simulink model "Device_B"  (R2025b)
settings: Solver=FixedStepAuto  StartTime=0.0  StopTime=10.0  RelTol=1e-3
undefined symbols (not defined in the file): bbb, Data_Display, Data_Display1, Data_Input2, Method_Select
libraries: androiduilib x4, dspxfrm3 x2, androidaudiovideolib x1, dspadpt3 x1, androidcommunicationlib x1
settings Model: Creator=chinm  LastModifiedBy=Windows
settings OptimizationCC: DefaultParameterBehavior=Inlined  EnhancedBackFolding=on  PassReuseOutputArgsAs=Individual arguments  ZeroExternalMemoryAtStartup=off  ZeroInternalMemoryAtStartup=off  MaxStackSize=64  OptimizeBlockOrder=speed  DifferentSizesBufferReuse=on  OptimizationCustomize=off  EfficientTunableParamExpr=on
settings DebuggingCC: ParameterTunabilityLossMsg=error
settings HardwareCC: ProdBitPerPointer=32.0  ProdBitPerSizeT=32.0  ProdBitPerPtrDiffT=32.0  ProdLargestAtomicInteger=Long  ProdLargestAtomicFloat=Double  ProdWordSize=32.0  ProdHWDeviceType=ARM Compatible->ARM Cortex-A (32-bit)
settings SFSimCC: MATLABDynamicMemAlloc=off
settings RTWCC: SystemTargetFile=ert.tlc  HardwareBoard=Android Device  TLCOptions="-aInlineSetEventsForThisBaseRateFcn=TLC_FALSE -aSuppressMultiTaskScheduler=TLC_FALSE  -aRateBasedStepFcn=0"  TemplateMakefile=ert_default_tmf  RTWVerbose=off  Toolchain=Android SDK/NDK Tools  GPUComputeCapability=3.5  Description=Embedded Coder
settings CodeAppCC: ForceParamTrailComments=on  IgnoreCustomStorageClasses=off  OperatorAnnotations=on  SimulinkDataObjDesc=on  SFDataObjDesc=on  InsertBlockDesc=on

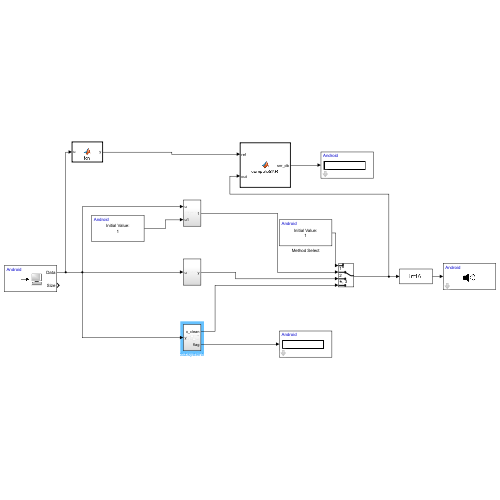
[thumbnail: Simulink's stored preview of the top-level diagram]
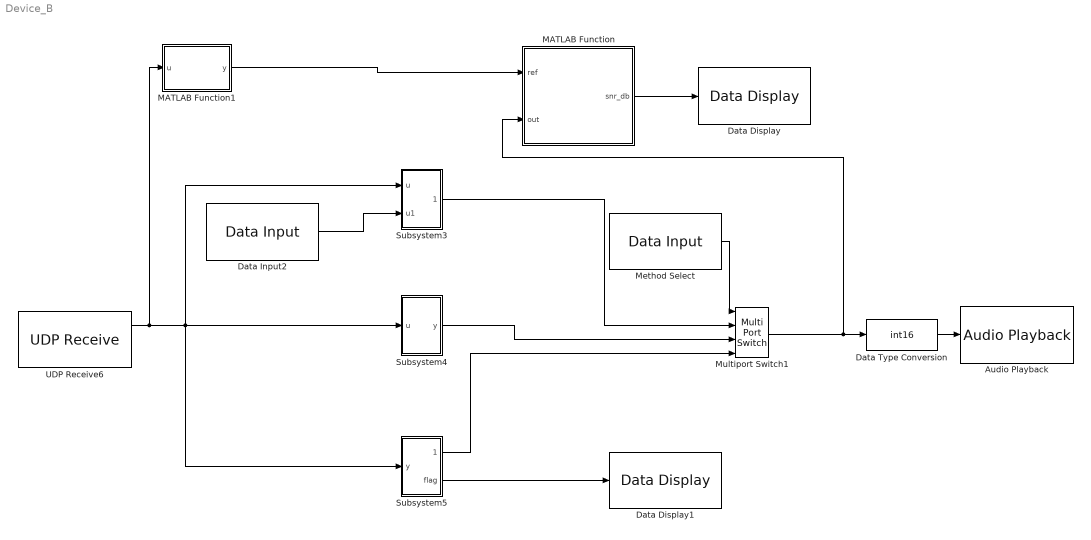
== system Device_B ==
  Audio Playback : androidaudiovideolib/Audio Playback  SampleFreq=8000  AudioSamplingFreq=8000  SampleTime=0.1  DeviceStr=0  QueueDuration=0  BlockPlatform=Android
  Data Display : androiduilib/Data Display  DataDisplayId=bbb/Data_Display  Format=Float  Precision=6  SimulateUsing=Code generation  blockPlatform=Android
  Data Display1 : androiduilib/Data Display  DataDisplayId=bbb/Data_Display1  Format=Float  Precision=6  SimulateUsing=Code generation  blockPlatform=Android
  Data Input2 : androiduilib/Data Input  isCharVector=off  Value=1.0  CharVector=Hello World  OutputDataType=int8  maxCharVectorSize=100  DataInputId=bbb/Data_Input2  SampleTime=1
  Data Type Conversion : DataTypeConversion  OutDataTypeStr=int16  SaturateOnIntegerOverflow=off  RndMeth=Floor
  MATLAB Function : MATLAB Function  TreatAsAtomicUnit=on
  MATLAB Function1 : MATLAB Function  TreatAsAtomicUnit=on
  Method Select : androiduilib/Data Input  isCharVector=off  Value=1  CharVector=Hello World  OutputDataType=int8  maxCharVectorSize=100  DataInputId=bbb/Method_Select  SampleTime=1
  Multiport Switch1 : MultiPortSwitch  DataPortOrder=Specify indices  OutDataTypeStr=double  SaturateOnIntegerOverflow=off  InputSameDT=off
  Subsystem3 : Subsystem
  Subsystem4 : Subsystem
  Subsystem5 : Subsystem
  UDP Receive6 : androidcommunicationlib/UDP Receive  localURL='0.0.0.0'  localPort=25070  remoteURL='0.0.0.0'  remotePort=-1  recvBufferSize=8192  signalDatatype=double  dims=1024  isVarSize=off  showBlockingTime=off  blockingTime=0  sampletime=0.032  blockPlatform=Android
  wires:
  Method Select/1 -> Multiport Switch1/1
  Data Input2/1 -> Subsystem3/2(u1)
  MATLAB Function/1(snr_db) -> Data Display/1
  Subsystem3/1(Out1) -> Multiport Switch1/2
  Multiport Switch1/1 -> MATLAB Function/2(out), Data Type Conversion/1
  UDP Receive6/1 -> MATLAB Function1/1(u), Subsystem4/1(u), Subsystem3/1(u), Subsystem5/1(y)
  Subsystem5/1(x_clean) -> Multiport Switch1/4
  Subsystem5/2(flag) -> Data Display1/1
  Subsystem4/1(y) -> Multiport Switch1/3
  MATLAB Function1/1(y) -> MATLAB Function/1(ref)
  Data Type Conversion/1 -> Audio Playback/1

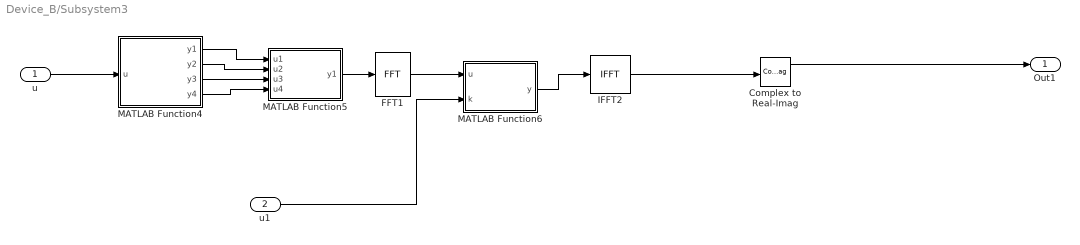
== system Device_B/Subsystem3 ==
  u : Inport
  u1 : Inport  Port=2
  Complex to Real-Imag : ComplexToRealImag
  FFT1 : dspxfrm3/FFT  FFTImplementation=Auto  CompMethod=Table lookup  TableOpt=NEW  TableOptActive=Speed  BitRevOrder=off  Normalize=off  InheritFFTLength=on  FFTLength=64  WrapInput=on  roundingMode=Ceiling  overflowMode=off  firstCoeffDataTypeStr=Inherit: Same word length as input  firstCoeffLastDataTypeStr=Inherit: Same word length as input  outputMin=[]  outputMax=[]
      settings: LockScale=on
  IFFT2 : dspxfrm3/IFFT  FFTImplementation=Auto  CompMethod=Table lookup  TableOpt=NEW  TableOptActive=Speed  BitRevOrder=off  cs_in=off  Normalize=on  InheritFFTLength=on  FFTLength=64  WrapInput=on  mode=Real  outSamplingMode=Sample based  roundingMode=Ceiling  overflowMode=off  firstCoeffDataTypeStr=Inherit: Same word length as input  firstCoeffLastDataTypeStr=Inherit: Same word length as input  outputMin=[]  outputMax=[]
  MATLAB Function4 : MATLAB Function  TreatAsAtomicUnit=on
  MATLAB Function5 : MATLAB Function  TreatAsAtomicUnit=on
  MATLAB Function6 : MATLAB Function  TreatAsAtomicUnit=on
  Out1 : Outport
  wires:
  Complex to Real-Imag/1 -> Out1/1
  IFFT2/1 -> Complex to Real-Imag/1
  MATLAB Function4/4(y4) -> MATLAB Function5/4(u4)
  u1/1 -> MATLAB Function6/2(k)
  MATLAB Function4/1(y1) -> MATLAB Function5/1(u1)
  MATLAB Function4/3(y3) -> MATLAB Function5/3(u3)
  MATLAB Function4/2(y2) -> MATLAB Function5/2(u2)
  MATLAB Function5/1(y1) -> FFT1/1
  MATLAB Function6/1(y) -> IFFT2/1
  u/1 -> MATLAB Function4/1(u)
  FFT1/1 -> MATLAB Function6/1(u)

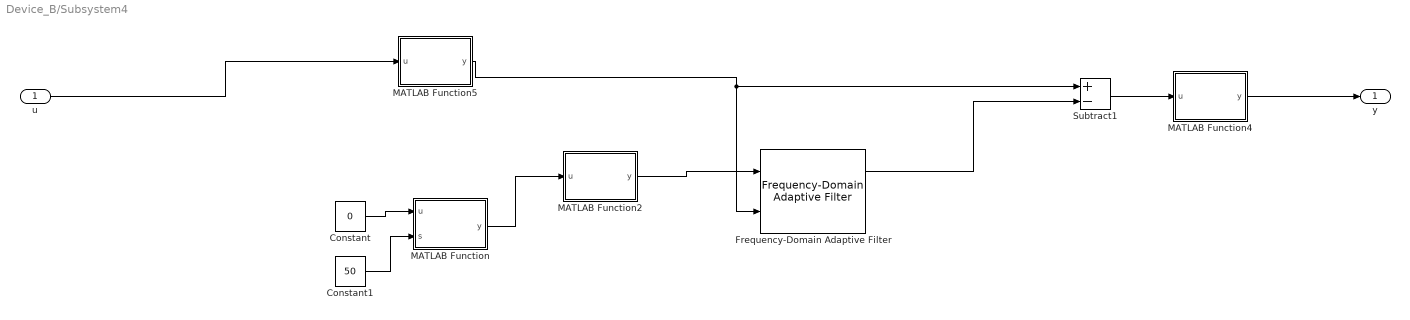
== system Device_B/Subsystem4 ==
  u : Inport
  Constant : Constant  Value=0  OutDataTypeStr=double
  Constant1 : Constant  Value=50
  Frequency-Domain Adaptive Filter : dspadpt3/Frequency-Domain Adaptive Filter  Method=Constrained FDAF  Length=32  BlockLength=32  StepSizePort=off  StepSize=1  LeakageFactorPort=off  LeakageFactor=1  AveragingFactorPort=off  AveragingFactor=0.9  OffsetPort=off  InitialPower=1  InitialCoefficients=0  AdaptPort=off  ResetPort=off  FFTCoefficientsPort=off  SimulateUsing=Interpreted execution  Offset=0
  MATLAB Function : MATLAB Function  TreatAsAtomicUnit=on
  MATLAB Function2 : MATLAB Function  TreatAsAtomicUnit=on
  MATLAB Function4 : MATLAB Function  TreatAsAtomicUnit=on
  MATLAB Function5 : MATLAB Function  TreatAsAtomicUnit=on
  Subtract1 : Sum  Inputs=+-
  y : Outport
  wires:
  MATLAB Function5/1(y) -> Frequency-Domain Adaptive Filter/2, Subtract1/1
  Subtract1/1 -> MATLAB Function4/1(u)
  Constant/1 -> MATLAB Function/1(u)
  MATLAB Function2/1(y) -> Frequency-Domain Adaptive Filter/1
  MATLAB Function/1(y) -> MATLAB Function2/1(u)
  Constant1/1 -> MATLAB Function/2(s)
  u/1 -> MATLAB Function5/1(u)
  MATLAB Function4/1(y) -> y/1
  Frequency-Domain Adaptive Filter/1 -> Subtract1/2

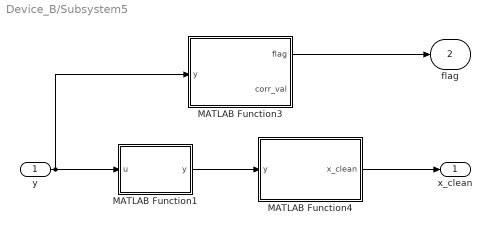
== system Device_B/Subsystem5 ==
  y : Inport
  MATLAB Function1 : MATLAB Function  TreatAsAtomicUnit=on
  MATLAB Function3 : MATLAB Function  TreatAsAtomicUnit=on
  MATLAB Function4 : MATLAB Function  TreatAsAtomicUnit=on
  x_clean : Outport
  flag : Outport  Port=2
  wires:
  y/1 -> MATLAB Function3/1(y), MATLAB Function1/1(u)
  MATLAB Function3/1(flag) -> flag/1
  MATLAB Function4/1(x_clean) -> x_clean/1
  MATLAB Function1/1(y) -> MATLAB Function4/1(y)

== matlab function Device_B/Subsystem5/MATLAB Function3 ==
  data: y input; flag output; corr_val output
function [flag, corr_val] = verify_watermark(y)

persistent key amp Fs watermark_freq watermark_phase
if isempty(key)
    key = 12345;
    amp = 0.05;
    Fs = 44100;
    watermark_freq = 100;
    watermark_phase = 2*pi * (key / 100000);
end

[N, C] = size(y);
corr_val = zeros(1, C);

t = (0:N-1)' / Fs;
w_ref = amp * sin(2*pi * watermark_freq * t + watermark_phase);

for c = 1:C
    correlation_matrix = corrcoef(y(:,c), w_ref);
    corr_val(c) = abs(correlation_matrix(1,2));
end

threshold = 0.1;
flag = any(corr_val > threshold);
end

== matlab function Device_B/MATLAB Function1 ==
  data: u input; y output
function y = fcn(u)
    y = randn(256,2);
    y(:,1) = u(1:256);
    y(:,2) = u(257:512);

== matlab function Device_B/Subsystem5/MATLAB Function1 ==
  data: u input; y output
function y = fcn(u)
    y = randn(256,2);
    y(:,1) = u(1:256);
    y(:,2) = u(257:512);

== matlab function Device_B/MATLAB Function ==
  data: ref input; snr_db output; out input
function snr_db = computeSNR(ref, out)
% ref and out are frame vectors of same size

noise = ref - out;

p_signal = sum(out.^2);
p_noise  = sum(noise.^2) + eps;

snr_db = -10*log10(p_signal / p_noise);
end

== matlab function Device_B/Subsystem5/MATLAB Function4 ==
  data: y input; x_clean output
function x_clean = remove_watermark(y)

persistent key amp Fs watermark_freq watermark_phase
if isempty(key)
    key = 12345;
    amp = 0.05;
    Fs = 44100;
    watermark_freq = 100;
    watermark_phase = 2*pi * (key / 100000);
end

[N, C] = size(y);
x_clean = zeros(N, C);

% Generate the watermark signal
t = (0:N-1)' / Fs;
w = amp * sin(2*pi * watermark_freq * t + watermark_phase);

% Remove watermark from each channel
for c = 1:C
    x_clean(:,c) = y(:,c) - w;
end

end

== matlab function Device_B/Subsystem4/MATLAB Function ==
  data: y output; u input double; s input
function y = fcn(u, s) 
y = s.*randn(256,2)+u;

== matlab function Device_B/Subsystem4/MATLAB Function2 ==
  data: u input; y output
function y = fcn(u)
y = randn(512,1);
y(1:256) = u(:,1);
y(257:512) = u(:,2);

== matlab function Device_B/Subsystem4/MATLAB Function4 ==
  data: u input; y output
function y = fcn(u)
y = randn(256,2);
y(:,1) =  u(1:256);
y(:,2) =  u(257:512);

== matlab function Device_B/Subsystem4/MATLAB Function5 ==
  data: u input; y output
function y = fcn(u)
y = randn(512,1);
y(1:512) = u(1:512);

== matlab function Device_B/Subsystem3/MATLAB Function4 ==
  data: u input; y1 output; y2 output; y3 output; y4 output
function [y1, y2, y3, y4] = fcn(u)
    y1 = u(1:256);
    y2 = u(257:512);
    y3 = u(513:768);
    y4 = u(769:1024);
    
end

== matlab function Device_B/Subsystem3/MATLAB Function5 ==
  data: u1 input; y1 output; u2 input; u3 input; u4 input
function y1 = fcn(u1,u2,u3,u4)
    y1 = [u1+1j*u3, u2+1j*u4];

end

== matlab function Device_B/Subsystem3/MATLAB Function6 ==
  data: u input; y output; k input
function y = descramble_stereo_fft(u, k)
    left_channel_scrambled = u(:, 1);
    right_channel_scrambled = u(:, 2);
    
    descrambled_left = descramble_channel(left_channel_scrambled, k);
    descrambled_right = descramble_channel(right_channel_scrambled, k);
    
    y = [descrambled_left, descrambled_right];
end

function descrambled_ch = descramble_channel(ch, k)
    N = length(ch);
    descrambled_ch = complex(zeros(N, 1));
    shift_amount = k*13;
    
    for i = 1:N
        new_i = mod(i - 1 - shift_amount, N) + 1;
        descrambled_ch(new_i) = ch(i);
    end
end
